simulink model "lab7_podwojne"  (R2024b)
settings: Solver=ode45  StartTime=0.0  StopTime=15.0  MaxStep=2^-5  RelTol=1e-3
settings Model: Creator=kg53848  LastModifiedBy=kg53848

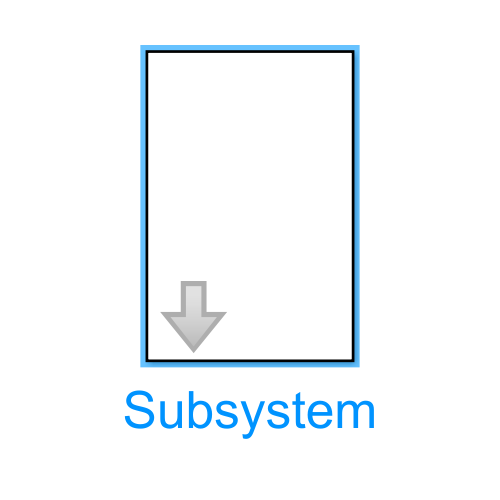
[thumbnail: Simulink's stored preview of the top-level diagram]
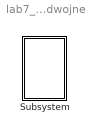
== system lab7_podwojne ==
  Subsystem : Subsystem  mask{g=9.81, k1=2, k2=1, m1=1, m2=2, l1=1, l2=2, fi10=80, fi20=150, fi11=0, fi21=0}
      mask prompts: g "przysp"; k1 "wsp tlum 1"; k2 "wsp tlum 2"; m1 "m wah 1"; m2 "m wah 2"; l1 "l 1"; l2 "l 2"; fi10 "kat wych wah 1"; fi20 "kat wych wah 2"; fi11 "V wah 1"; fi21 "V wah 2"

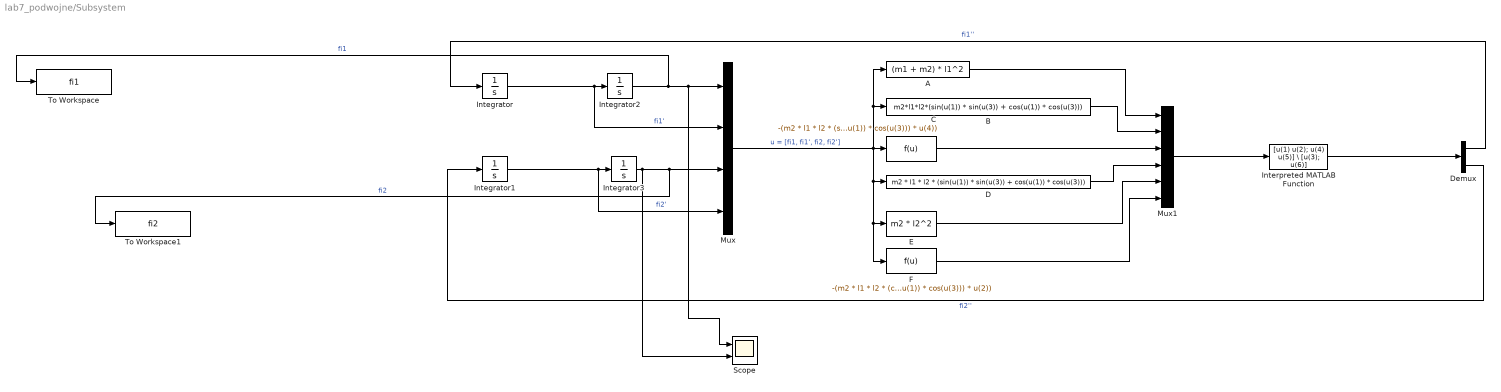
== system lab7_podwojne/Subsystem ==
  A : Fcn  Expr=(m1 + m2) * l1^2
  B : Fcn  Expr=m2*l1*l2*(sin(u(1)) * sin(u(3)) + cos(u(1)) * cos(u(3)))
  C : Fcn  Expr=-(m2 * l1 * l2 * (sin(u(1)) * cos(u(3)) - cos(u(1)) * sin(u(3))) * u(4)^2 + (m1 + m2) * g * l1 * sin(u(1)) + k1 * l1^2 * u(2) + k2 * l1 * l2 * (sin(u(1)) * sin(u(3)) + cos(u(1)) * cos(u(3))) * u(4))
  D : Fcn  Expr=m2 * l1 * l2 * (sin(u(1)) * sin(u(3)) + cos(u(1)) * cos(u(3)))
  Demux : Demux  Outputs=2
  E : Fcn  Expr=m2 * l2^2
  F : Fcn  Expr=-(m2 * l1 * l2 * (cos(u(1)) * sin(u(3)) - sin(u(1)) * cos(u(3))) * u(2)^2 + m2 * g * l2 * sin(u(3)) + k2 * l2^2 * u(4) + k2 * l1 * l2 *(sin(u(1)) * sin(u(3)) + cos(u(1)) * cos(u(3))) * u(2))
  Integrator : Integrator  InitialCondition=fi11 * pi/180
  Integrator1 : Integrator  InitialCondition=fi21 * pi/180
  Integrator2 : Integrator  InitialCondition=fi10 * pi/180
  Integrator3 : Integrator  InitialCondition=fi20 * pi/180
  Interpreted MATLAB Function : MATLABFcn  MATLABFcn=[u(1) u(2); u(4) u(5)] \ [u(3); u(6)]
  Mux : Mux
  Mux1 : Mux  Inputs=6
  Scope : Scope  NumInputPorts=2
  To Workspace : ToWorkspace  VariableName=fi1  SampleTime=-1
  To Workspace1 : ToWorkspace  VariableName=fi2  SampleTime=-1
  wires:
  Demux/2 -> Integrator1/1  "fi2''"
  E/1 -> Mux1/5
  Mux/1 -> F/1, E/1, D/1, B/1, A/1, C/1  "u = [fi1, fi1', fi2, fi2']"
  Integrator2/1 -> To Workspace/1, Mux/1, Scope/1  "fi1"
  B/1 -> Mux1/2
  Integrator1/1 -> Mux/4, Integrator3/1  "fi2'"
  D/1 -> Mux1/4
  Integrator/1 -> Mux/2, Integrator2/1  "fi1'"
  Integrator3/1 -> To Workspace1/1, Mux/3, Scope/2  "fi2"
  F/1 -> Mux1/6
  Demux/1 -> Integrator/1  "fi1''"
  A/1 -> Mux1/1
  C/1 -> Mux1/3
  Interpreted MATLAB Function/1 -> Demux/1
  Mux1/1 -> Interpreted MATLAB Function/1
